simulink model "HighPass_Sim"  (R2022b)
settings: Solver=VariableStepAuto  StartTime=0.0  StopTime=1  RelTol=1e-3
values from neighbouring files (symbols this model uses):
  amplitude_input = 1    [HP_config.m]
  denGs = [1 wc]    [HP_config.m]
  denGz = cell2mat(Gz.Denominator)    [HP_config.m]
  numGs = [1 wc/10]    [HP_config.m]
  numGz = cell2mat(Gz.Numerator)    [HP_config.m]
  offset_input = 0    [HP_config.m]
  Ts = 1/f_sample    (= 1.42857142857e-05)    [HP_config.m]
  Tsim = 0.1*Ts    (= 1.42857142857e-06)    [HP_config.m]
  w_input = 2*pi*f_input    (= 62.8318530718)    [HP_config.m]
settings Model: Creator=mluser  LastModifiedBy=mluser
settings SFSimCC: SimCustomHeaderCode="#include \"HighPass.h\""  SimUserSources=HighPass.c  SimUserIncludeDirs=MATLAB Drive/Regulacion/Filtros/HighPass
settings RTWCC: RTWUseSimCustomCode=on  CustomHeaderCode="#include \"HighPass.h\""  CustomInclude=MATLAB Drive/Regulacion/Filtros/HighPass  CustomSource=HighPass.c

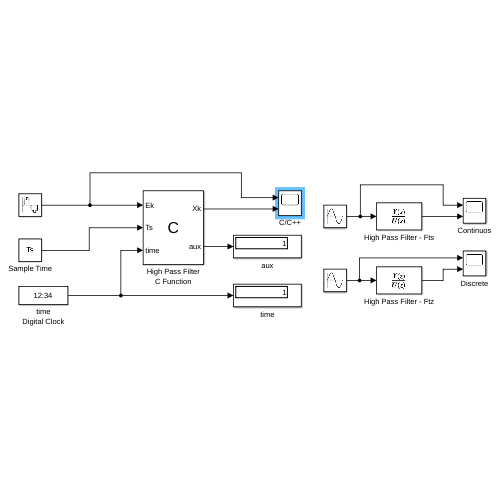
[thumbnail: Simulink's stored preview of the top-level diagram]
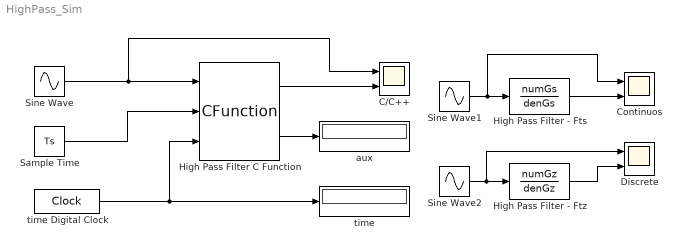
== system HighPass_Sim ==
  C/C++ : Scope  NumInputPorts=2
  Continuos : Scope  NumInputPorts=2
  Discrete : Scope  NumInputPorts=2
  High Pass Filter C Function : CFunction  OutputCode=Xk=HighPass(Ek, Ts, time, &aux);
  High Pass Filter - Fts : TransferFcn  Numerator=numGs  Denominator=denGs
  High Pass Filter - Ftz : DiscreteTransferFcn  Numerator=numGz  Denominator=denGz
  Sample Time : Constant  Value=Ts
  Sine Wave : Sin  Amplitude=amplitude_input  Bias=offset_input  Frequency=w_input  SampleTime=Tsim
  Sine Wave1 : Sin  Amplitude=amplitude_input  Bias=offset_input  Frequency=w_input  SampleTime=0
  Sine Wave2 : Sin  Amplitude=amplitude_input  Bias=offset_input  Frequency=w_input  SampleTime=0
  aux : Display
  time : Display
  time Digital Clock : DigitalClock  SampleTime=Tsim
  wires:
  Sine Wave/1 -> C/C++/1, High Pass Filter C Function/1
  Sample Time/1 -> High Pass Filter C Function/2
  time Digital Clock/1 -> time/1, High Pass Filter C Function/3
  High Pass Filter C Function/1 -> C/C++/2
  Sine Wave1/1 -> Continuos/1, High Pass Filter - Fts/1
  High Pass Filter C Function/2 -> aux/1
  Sine Wave2/1 -> Discrete/1, High Pass Filter - Ftz/1
  High Pass Filter - Fts/1 -> Continuos/2
  High Pass Filter - Ftz/1 -> Discrete/2
